simulink model "UAV3atitude_int"  (R2024b)
settings: Solver=VariableStepAuto  StartTime=0.0  StopTime=tsim  RelTol=1e-3
values from neighbouring files (symbols this model uses):
  A = [ybb, yp+(w0/u0), yr-(u0/u0), g*cos(tt0)/u0 ... (first row only)    [init.m]    (also in new_A_B_integrativos.m = [A, zeros, zeros]; new_A_B_lambda.m = [A, zeros])
  B = [Yda, Ydr ... (first row only)    [init.m]    (also in new_A_B_integrativos.m = [B; new_line_bb; new_line_lambda]; new_A_B_lambda.m = [B; new_line_B])
  C = [1,0,0,0,0 ... (first row only)    [main.m]    (also in untitled2.m = diag([1,1,1,1]))
  D = zeros(2,2)    [main.m]    (also in untitled2.m = zeros(4,2))
  K = lqr(A_temp,B_temp,Q,R)    [K_lqr.m]    (also in k_finder.m = [0,0,0,0; main.m; untitled2.m = [0,0,0.229,0])
  r = [deg2rad(10), deg2rad(20)]    [main.m]
  x0 = min(y_diff.signals.values)    [graficos_formacao.m]    (also in init.m = [0,0,0,0]; new_A_B_lambda.m = [0,0,0,0,0]')
settings Model: Creator=ruben  LastModifiedBy=ruben
settings DataIOCC: ReturnWorkspaceOutputs=off
settings DebuggingCC: AlgebraicLoopMsg=none

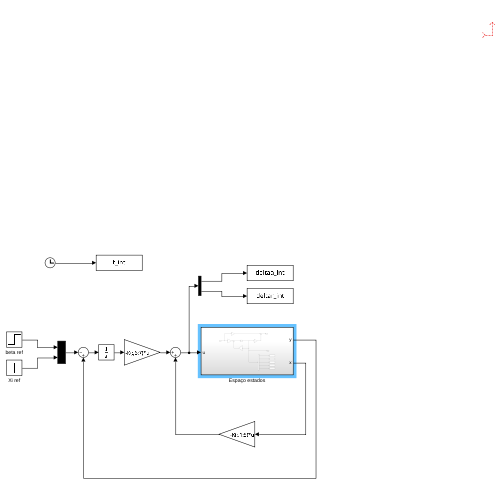
[thumbnail: Simulink's stored preview of the top-level diagram]
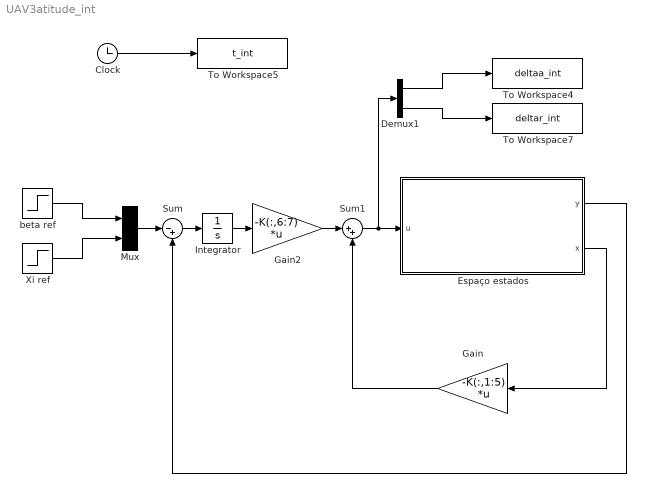
== system UAV3atitude_int ==
  Clock : Clock
  Demux1 : Demux  Outputs=2
  Espaço estados : Subsystem
  Gain : Gain  Gain=-K(:,1:5)  Multiplication=Matrix(K*u)
  Gain2 : Gain  Gain=-K(:,6:7)  Multiplication=Matrix(K*u)
  Integrator : Integrator  InitialCondition=[0,0]
  Mux : Mux  Inputs=2
  Sum : Sum  Inputs=|-+
  Sum1 : Sum  Inputs=|++
  To Workspace4 : ToWorkspace  VariableName=deltaa_int  SampleTime=-1
  To Workspace5 : ToWorkspace  VariableName=t_int  SampleTime=-1
  To Workspace7 : ToWorkspace  VariableName=deltar_int  SampleTime=-1
  Xi ref : Step  After=r(2)  SampleTime=0
  beta ref : Step  After=r(1)  SampleTime=0
  wires:
  Demux1/1 -> To Workspace4/1
  Demux1/2 -> To Workspace7/1
  Clock/1 -> To Workspace5/1
  beta ref/1 -> Mux/1
  Xi ref/1 -> Mux/2
  ? -> ?
  Espaço estados/2(x) -> Gain/1
  Mux/1 -> Sum/1
  Espaço estados/1(y) -> Sum/2
  Sum1/1 -> Demux1/1, Espaço estados/1(u)
  Gain/1 -> Sum1/2
  Integrator/1 -> Gain2/1
  Sum/1 -> Integrator/1
  Gain2/1 -> Sum1/1

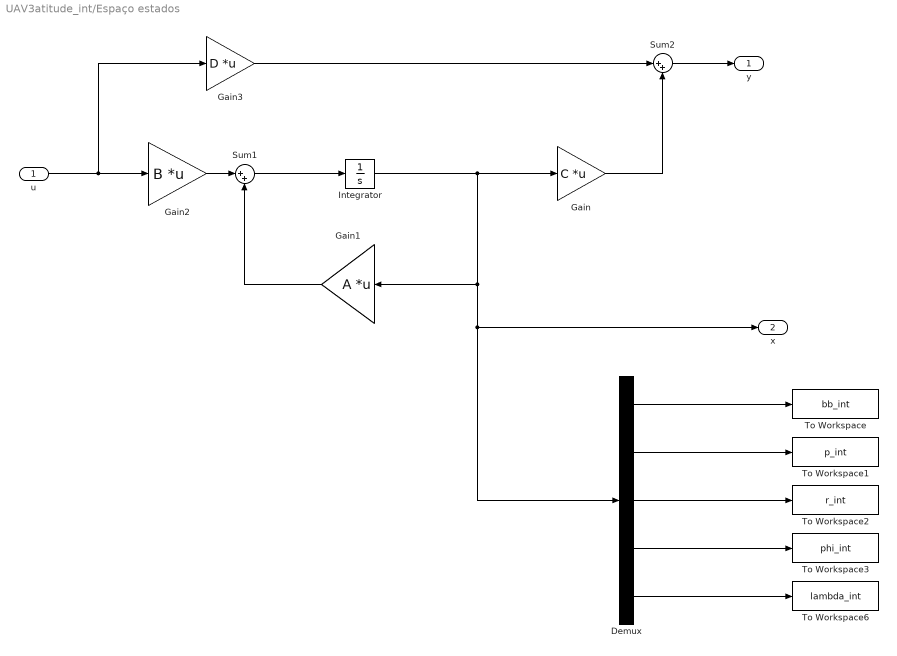
== system UAV3atitude_int/Espaço estados ==
  u : Inport
  Demux : Demux  Outputs=5
  Gain : Gain  Gain=C  Multiplication=Matrix(K*u)
  Gain1 : Gain  Gain=A  Multiplication=Matrix(K*u)
  Gain2 : Gain  Gain=B  Multiplication=Matrix(K*u)
  Gain3 : Gain  Gain=D  Multiplication=Matrix(K*u)
  Integrator : Integrator  InitialCondition=x0
  Sum1 : Sum  Inputs=|++
  Sum2 : Sum  Inputs=|++
  To Workspace : ToWorkspace  VariableName=bb_int  SampleTime=-1
  To Workspace1 : ToWorkspace  VariableName=p_int  SampleTime=-1
  To Workspace2 : ToWorkspace  VariableName=r_int  SampleTime=-1
  To Workspace3 : ToWorkspace  VariableName=phi_int  SampleTime=-1
  To Workspace6 : ToWorkspace  VariableName=lambda_int  SampleTime=-1
  y : Outport
  x : Outport  Port=2
  wires:
  u/1 -> Gain3/1, Gain2/1
  Sum1/1 -> Integrator/1
  Demux/4 -> To Workspace3/1
  Demux/3 -> To Workspace2/1
  Demux/1 -> To Workspace/1
  Demux/2 -> To Workspace1/1
  Demux/5 -> To Workspace6/1
  Gain2/1 -> Sum1/1
  Integrator/1 -> Gain1/1, x/1, Demux/1, Gain/1
  Gain1/1 -> Sum1/2
  Gain/1 -> Sum2/2
  Gain3/1 -> Sum2/1
  Sum2/1 -> y/1
